simulink model "DriverRequest"  (R2021b)
settings: configuration reference "csSingleInstance" (kept outside this file)
undefined symbols (not defined in the file or in its folder): reqMode
libraries: simulink x20
Description:
  | This is the base model from which the ISO model template is derived.
settings Model: DataDictionary=DD_DriverRequest.sldd  EnableAccessToBaseWorkspace=off  Creator=rsnah  LastModifiedBy=rsnah
settings ConfigSetRef: SourceName=csSingleInstance

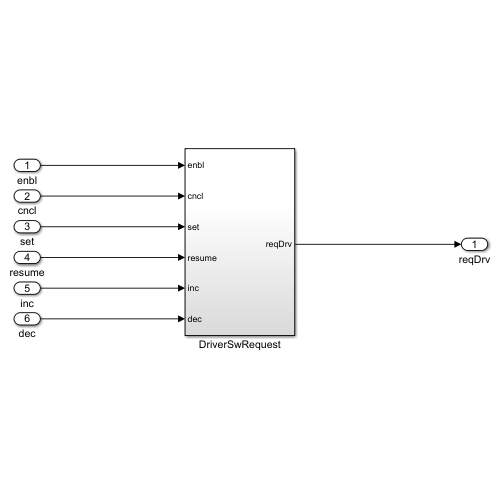
[thumbnail: Simulink's stored preview of the top-level diagram]
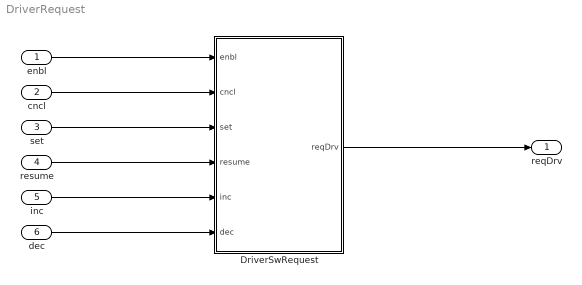
== system DriverRequest ==
  enbl : Inport  OutDataTypeStr=boolean  PortDimensions=1  SampleTime=0.01
  cncl : Inport  Port=2  OutDataTypeStr=boolean  PortDimensions=1  SampleTime=0.01
  set : Inport  Port=3  OutDataTypeStr=boolean  PortDimensions=1  SampleTime=0.01
  resume : Inport  Port=4  OutDataTypeStr=boolean  PortDimensions=1  SampleTime=0.01
  inc : Inport  Port=5  OutDataTypeStr=boolean  PortDimensions=1  SampleTime=0.01
  dec : Inport  Port=6  OutDataTypeStr=boolean  PortDimensions=1  SampleTime=0.01
  DriverSwRequest : Subsystem
  reqDrv : Outport  VectorParamsAs1DForOutWhenUnconnected=off
  wires:
  enbl/1 -> DriverSwRequest/1(enbl)
  dec/1 -> DriverSwRequest/6(dec)
  inc/1 -> DriverSwRequest/5(inc)
  resume/1 -> DriverSwRequest/4(resume)
  cncl/1 -> DriverSwRequest/2(cncl)
  set/1 -> DriverSwRequest/3(set)
  DriverSwRequest/1(reqDrv) -> reqDrv/1

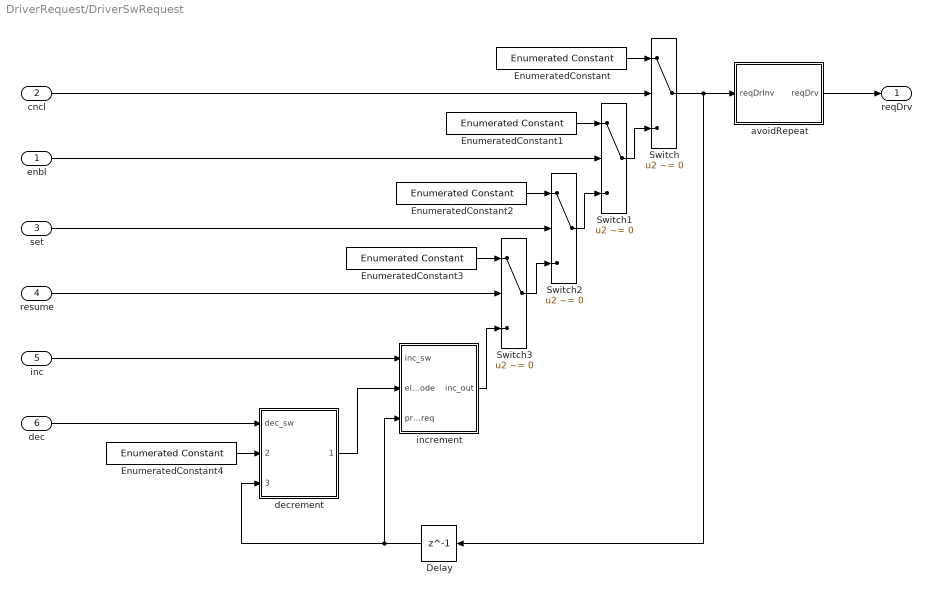
== system DriverRequest/DriverSwRequest ==
  enbl : Inport
  cncl : Inport  Port=2
  set : Inport  Port=3
  resume : Inport  Port=4
  inc : Inport  Port=5  OutDataTypeStr=boolean
  dec : Inport  Port=6  OutDataTypeStr=boolean
  Delay : Delay  DelayLength=1  InitialCondition=reqMode.NoRequest
      settings: AttributesFormatString=IC: %<InitialCondition>
  EnumeratedConstant : simulink/Sources/Enumerated Constant  OutDataTypeStr=Enum: reqMode  Value=reqMode.Cancel  SampleTime=inf
  EnumeratedConstant1 : simulink/Sources/Enumerated Constant  OutDataTypeStr=Enum: reqMode  Value=reqMode.Cruise  SampleTime=inf
  EnumeratedConstant2 : simulink/Sources/Enumerated Constant  OutDataTypeStr=Enum: reqMode  Value=reqMode.Set  SampleTime=inf
  EnumeratedConstant3 : simulink/Sources/Enumerated Constant  OutDataTypeStr=Enum: reqMode  Value=reqMode.ResumeReq  SampleTime=inf
  EnumeratedConstant4 : simulink/Sources/Enumerated Constant  OutDataTypeStr=Enum: reqMode  Value=reqMode.NoRequest  SampleTime=inf
  Switch{,1..3} (4 alike) : Switch  Criteria=u2 ~= 0
  avoidRepeat : Subsystem
  decrement : Subsystem
  increment : Subsystem
  reqDrv : Outport  VectorParamsAs1DForOutWhenUnconnected=off
  wires:
  EnumeratedConstant/1 -> Switch/1
  Switch/1 -> Delay/1, avoidRepeat/1(reqDrInv)
  cncl/1 -> Switch/2
  enbl/1 -> Switch1/2
  EnumeratedConstant1/1 -> Switch1/1
  Switch1/1 -> Switch/3
  set/1 -> Switch2/2
  EnumeratedConstant2/1 -> Switch2/1
  resume/1 -> Switch3/2
  EnumeratedConstant3/1 -> Switch3/1
  Switch3/1 -> Switch2/3
  Switch2/1 -> Switch1/3
  dec/1 -> decrement/1(dec_sw)
  EnumeratedConstant4/1 -> decrement/2(else_mode)
  inc/1 -> increment/1(inc_sw)
  decrement/1(dec_out) -> increment/2(else_mode)
  increment/1(inc_out) -> Switch3/3
  Delay/1 -> increment/3(prev_req), decrement/3(prev_req)
  avoidRepeat/1(reqDrv) -> reqDrv/1

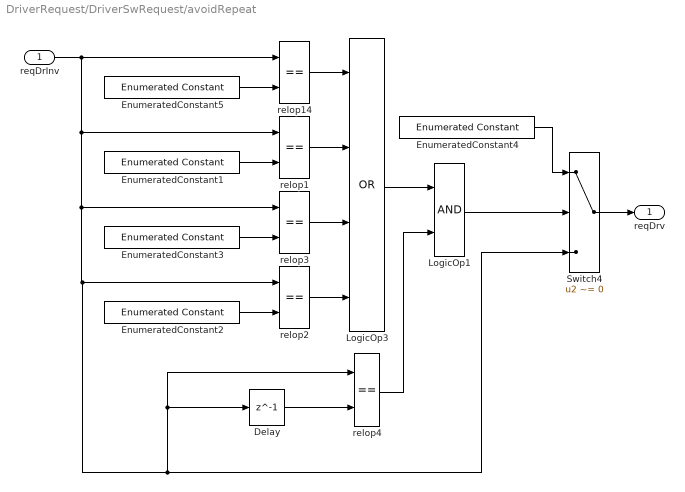
== system DriverRequest/DriverSwRequest/avoidRepeat ==
  reqDrInv : Inport
  Delay : Delay  DelayLength=1  InitialCondition=reqMode.NoRequest
      settings: AttributesFormatString=Init = %<InitialCondition>
  EnumeratedConstant1 : simulink/Sources/Enumerated Constant  OutDataTypeStr=Enum: reqMode  Value=reqMode.Cruise  SampleTime=inf
  EnumeratedConstant2 : simulink/Sources/Enumerated Constant  OutDataTypeStr=Enum: reqMode  Value=reqMode.ResumeReq  SampleTime=inf
  EnumeratedConstant3 : simulink/Sources/Enumerated Constant  OutDataTypeStr=Enum: reqMode  Value=reqMode.Set  SampleTime=inf
  EnumeratedConstant4 : simulink/Sources/Enumerated Constant  OutDataTypeStr=Enum: reqMode  Value=reqMode.NoRequest  SampleTime=inf
  EnumeratedConstant5 : simulink/Sources/Enumerated Constant  OutDataTypeStr=Enum: reqMode  Value=reqMode.Cancel  SampleTime=inf
  LogicOp1 : Logic  AllPortsSameDT=off  OutDataTypeStr=boolean
  LogicOp3 : Logic  Operator=OR  Inputs=4  AllPortsSameDT=off  OutDataTypeStr=boolean
  Switch4 : Switch  Criteria=u2 ~= 0
  relop{1..4,14} (5 alike) : RelationalOperator  Operator===  OutDataTypeStr=boolean  RndMeth=Nearest
  reqDrv : Outport  VectorParamsAs1DForOutWhenUnconnected=off
  wires:
  EnumeratedConstant5/1 -> relop14/2
  EnumeratedConstant1/1 -> relop1/2
  EnumeratedConstant3/1 -> relop3/2
  EnumeratedConstant2/1 -> relop2/2
  reqDrInv/1 -> Switch4/3, relop4/1, Delay/1, relop2/1, relop3/1, relop1/1, relop14/1
  relop14/1 -> LogicOp3/1
  relop1/1 -> LogicOp3/2
  relop3/1 -> LogicOp3/3
  relop2/1 -> LogicOp3/4
  Switch4/1 -> reqDrv/1
  Delay/1 -> relop4/2
  relop4/1 -> LogicOp1/2
  LogicOp3/1 -> LogicOp1/1
  LogicOp1/1 -> Switch4/2
  EnumeratedConstant4/1 -> Switch4/1

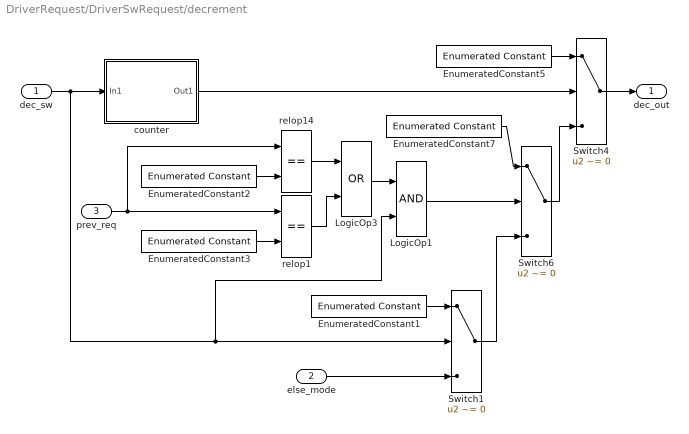
== system DriverRequest/DriverSwRequest/decrement ==
  dec_sw : Inport
  else_mode : Inport  Port=2
  prev_req : Inport  Port=3
  EnumeratedConstant1 : simulink/Sources/Enumerated Constant  OutDataTypeStr=Enum: reqMode  Value=reqMode.Dec_Short  SampleTime=inf
  EnumeratedConstant2 : simulink/Sources/Enumerated Constant  OutDataTypeStr=Enum: reqMode  Value=reqMode.Dec_Short  SampleTime=inf
  EnumeratedConstant3 : simulink/Sources/Enumerated Constant  OutDataTypeStr=Enum: reqMode  Value=reqMode.Dec_Middle  SampleTime=inf
  EnumeratedConstant5 : simulink/Sources/Enumerated Constant  OutDataTypeStr=Enum: reqMode  Value=reqMode.Dec_Long  SampleTime=inf
  EnumeratedConstant7 : simulink/Sources/Enumerated Constant  OutDataTypeStr=Enum: reqMode  Value=reqMode.Dec_Middle  SampleTime=inf
  LogicOp1 : Logic  AllPortsSameDT=off  OutDataTypeStr=boolean
  LogicOp3 : Logic  Operator=OR  AllPortsSameDT=off  OutDataTypeStr=boolean
  Switch1 : Switch  Criteria=u2 ~= 0
  Switch4 : Switch  Criteria=u2 ~= 0
  Switch6 : Switch  Criteria=u2 ~= 0
  counter : Subsystem  DisableCoverage=on  mask(SLDV counter){CountValue=50, OutDataTypeStr=uint8}
      mask prompts: CountValue "Count value"; OutDataTypeStr "Data type"
      mask help: A counter block optimized for Simulink Design Verifier test case generation. If the input is true for consecutive steps which is specified the Count value parameter, then the output is TRUE, otherwise it is FALSE.
      mask init:
      | if CountValue < 0 || CountValue > intmax(OutDataTypeStr)
      |     error('Specified count value needs to be within 0-%d.',intmax(OutDataTypeStr))
      | end
      mask Display: disp(sprintf('Counter (%s)\nCount:%d',OutDataTypeStr,CountValue))
  relop1 : RelationalOperator  Operator===  OutDataTypeStr=boolean  RndMeth=Nearest
  relop14 : RelationalOperator  Operator===  OutDataTypeStr=boolean  RndMeth=Nearest
  dec_out : Outport  VectorParamsAs1DForOutWhenUnconnected=off
  wires:
  EnumeratedConstant5/1 -> Switch4/1
  Switch4/1 -> dec_out/1
  EnumeratedConstant7/1 -> Switch6/1
  Switch6/1 -> Switch4/3
  counter/1(Out1) -> Switch4/2
  Switch1/1 -> Switch6/3
  dec_sw/1 -> counter/1(In1), LogicOp1/2, Switch1/2
  else_mode/1 -> Switch1/3
  EnumeratedConstant1/1 -> Switch1/1
  EnumeratedConstant2/1 -> relop14/2
  EnumeratedConstant3/1 -> relop1/2
  prev_req/1 -> relop14/1, relop1/1
  relop14/1 -> LogicOp3/1
  relop1/1 -> LogicOp3/2
  LogicOp3/1 -> LogicOp1/1
  LogicOp1/1 -> Switch6/2

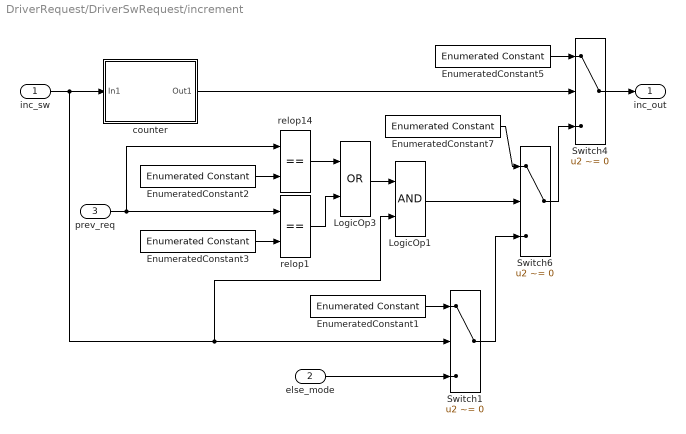
== system DriverRequest/DriverSwRequest/increment ==
  inc_sw : Inport
  else_mode : Inport  Port=2
  prev_req : Inport  Port=3
  EnumeratedConstant1 : simulink/Sources/Enumerated Constant  OutDataTypeStr=Enum: reqMode  Value=reqMode.Inc_Short  SampleTime=inf
  EnumeratedConstant2 : simulink/Sources/Enumerated Constant  OutDataTypeStr=Enum: reqMode  Value=reqMode.Inc_Short  SampleTime=inf
  EnumeratedConstant3 : simulink/Sources/Enumerated Constant  OutDataTypeStr=Enum: reqMode  Value=reqMode.Inc_Middle  SampleTime=inf
  EnumeratedConstant5 : simulink/Sources/Enumerated Constant  OutDataTypeStr=Enum: reqMode  Value=reqMode.Inc_Long  SampleTime=inf
  EnumeratedConstant7 : simulink/Sources/Enumerated Constant  OutDataTypeStr=Enum: reqMode  Value=reqMode.Inc_Middle  SampleTime=inf
  LogicOp1 : Logic  AllPortsSameDT=off  OutDataTypeStr=boolean
  LogicOp3 : Logic  Operator=OR  AllPortsSameDT=off  OutDataTypeStr=boolean
  Switch1 : Switch  Criteria=u2 ~= 0
  Switch4 : Switch  Criteria=u2 ~= 0
  Switch6 : Switch  Criteria=u2 ~= 0
  counter : Subsystem  DisableCoverage=on  mask(SLDV counter){CountValue=50, OutDataTypeStr=uint8}
      mask prompts: CountValue "Count value"; OutDataTypeStr "Data type"
      mask help: A counter block optimized for Simulink Design Verifier test case generation. If the input is true for consecutive steps which is specified the Count value parameter, then the output is TRUE, otherwise it is FALSE.
      mask init:
      | if CountValue < 0 || CountValue > intmax(OutDataTypeStr)
      |     error('Specified count value needs to be within 0-%d.',intmax(OutDataTypeStr))
      | end
      mask Display: disp(sprintf('Counter (%s)\nCount:%d',OutDataTypeStr,CountValue))
  relop1 : RelationalOperator  Operator===  OutDataTypeStr=boolean  RndMeth=Nearest
  relop14 : RelationalOperator  Operator===  OutDataTypeStr=boolean  RndMeth=Nearest
  inc_out : Outport  VectorParamsAs1DForOutWhenUnconnected=off
  wires:
  EnumeratedConstant5/1 -> Switch4/1
  Switch4/1 -> inc_out/1
  EnumeratedConstant7/1 -> Switch6/1
  Switch6/1 -> Switch4/3
  counter/1(Out1) -> Switch4/2
  Switch1/1 -> Switch6/3
  inc_sw/1 -> counter/1(In1), LogicOp1/2, Switch1/2
  else_mode/1 -> Switch1/3
  EnumeratedConstant1/1 -> Switch1/1
  EnumeratedConstant2/1 -> relop14/2
  EnumeratedConstant3/1 -> relop1/2
  prev_req/1 -> relop14/1, relop1/1
  relop14/1 -> LogicOp3/1
  relop1/1 -> LogicOp3/2
  LogicOp3/1 -> LogicOp1/1
  LogicOp1/1 -> Switch6/2

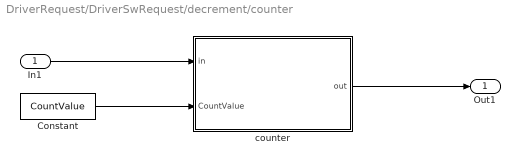
== system DriverRequest/DriverSwRequest/decrement/counter ==
  In1 : Inport
  Constant : Constant  Value=CountValue  OutDataTypeStr=OutDataTypeStr
  counter : MATLAB Function  TreatAsAtomicUnit=on
  Out1 : Outport  VectorParamsAs1DForOutWhenUnconnected=off
  wires:
  Constant/1 -> counter/2(CountValue)
  counter/1(out) -> Out1/1
  In1/1 -> counter/1(in)

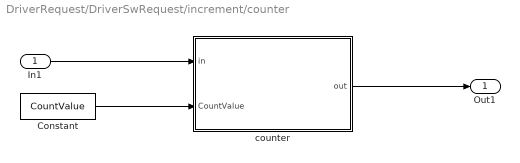
== system DriverRequest/DriverSwRequest/increment/counter ==
  In1 : Inport
  Constant : Constant  Value=CountValue  OutDataTypeStr=OutDataTypeStr
  counter : MATLAB Function  TreatAsAtomicUnit=on
  Out1 : Outport  VectorParamsAs1DForOutWhenUnconnected=off
  wires:
  Constant/1 -> counter/2(CountValue)
  counter/1(out) -> Out1/1
  In1/1 -> counter/1(in)

== matlab function DriverRequest/DriverSwRequest/increment/counter/counter ==
  data: in input boolean size=1; out output boolean size=1; CountValue input uint8 size=1
function out = counter(in,CountValue)
% DESCRIPTION:
%   Counter to limit.
%
% INPUT(S):
%   in - Enable the counter if true.
%   CountValue - Counter limit.
%
% OUTPUT(S):
%   out - Return true when counter limit is hit, false otherwise.

%#codegen

persistent cnt;

% initialize
if isempty(cnt)
    cnt = cast(0,'like',CountValue);
end

% if enabled
if in
    % Output true if CountValue is reached
    if cnt >= CountValue
        out = true;
    else
        % Continue counting up and output false
        cnt = cnt + cast(1,'like',CountValue);
        out = false;
    end
else
    % if disabled, output false and reset
    cnt = cast(0,'like',CountValue);
    out = false;
end

== matlab function DriverRequest/DriverSwRequest/decrement/counter/counter ==
  data: in input boolean size=1; out output boolean size=1; CountValue input uint8 size=1
function out = counter(in,CountValue)
% DESCRIPTION:
%   Counter to limit.
%
% INPUT(S):
%   in - Enable the counter if true.
%   CountValue - Counter limit.
%
% OUTPUT(S):
%   out - Return true when counter limit is hit, false otherwise.

%#codegen

persistent cnt;

% initialize
if isempty(cnt)
    cnt = cast(0,'like',CountValue);
end

% if enabled
if in
    % Output true if CountValue is reached
    if cnt >= CountValue
        out = true;
    else
        % Continue counting and output false        
        cnt = cnt + cast(1,'like',CountValue);
        out = false;
    end
else
    % if disabled, output false and reset
    cnt = cast(0,'like',CountValue);
    out = false;
end
